simulink model "Parallel_Force_Position_Control"  (R2020b)
settings: Solver=VariableStepAuto  StartTime=0.0  StopTime=20  RelTol=1e-3
values from neighbouring files (symbols this model uses):
  B = myRobot.B_Lagrangian    [hw15_main.m]
  C = myRobot.C_Lagrangian    [hw15_main.m]
  dJ = dJ(1:3  ,:)    [hw15_main.m]
  F = myRobot.F    [hw15_main.m]
  fd = [0;1;0]    [hw15_main.m]
  G = myRobot.G_Lagrangian    [hw15_main.m]
  J_inv = pinv(J)    [hw15_main.m]
  Ja = Ja(1:3,:)    [hw15_main.m]
  K = diag([1 1 1])    [hw15_main.m]
  Kd = diag([1 20 1])    [hw15_main.m]
  Kf = diag([1 10 1]).*10    [hw15_main.m]
  Ki = diag([1 10 1])    [hw15_main.m]
  Kp = diag([1 0.5 1])    [hw15_main.m]
  Md = diag([1 1 1])    [hw15_main.m]
  Md_inv = pinv(Md)    [hw15_main.m]
  xd = [0.3;0;0.1]    [hw15_main.m]
  xr = [0;0.3;0]    [hw15_main.m]
settings Model: Creator=nicol  LastModifiedBy=nicol

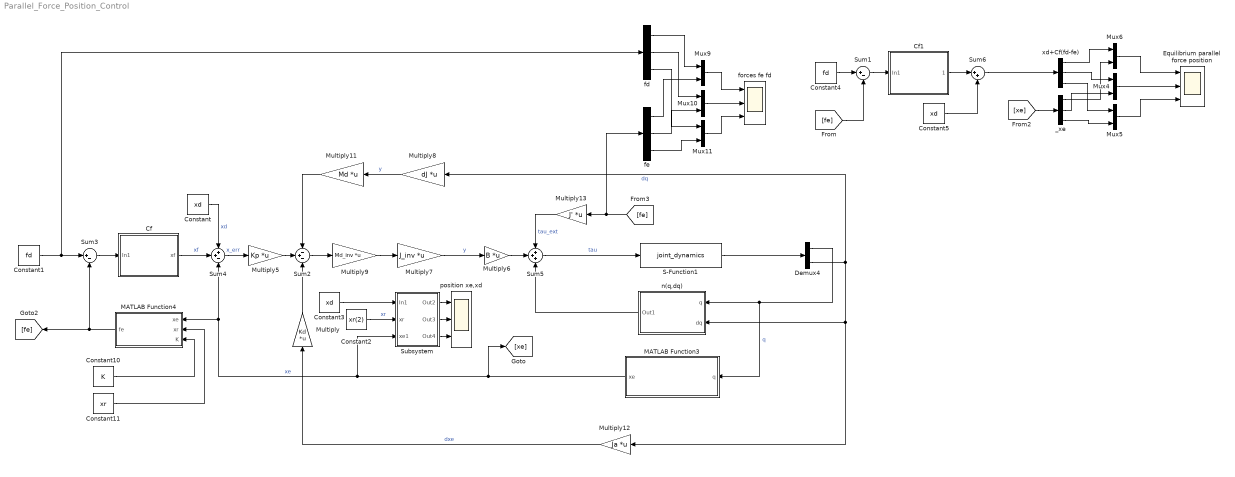
== system Parallel_Force_Position_Control ==
  Cf : Subsystem
  Cf1 : Subsystem
  Constant : Constant  Value=xd
  Constant1 : Constant  Value=fd
  Constant10 : Constant  Value=K
  Constant11 : Constant  Value=xr
  Constant2 : Constant  Value=xr(2)
  Constant3 : Constant  Value=xd
  Constant4 : Constant  Value=fd
  Constant5 : Constant  Value=xd
  Demux4 : Demux  Outputs=2
  Equilibrium parallel force position : Scope  NumInputPorts=3
  MATLAB Function3 : MATLAB Function  TreatAsAtomicUnit=on
  MATLAB Function4 : MATLAB Function  TreatAsAtomicUnit=on
  Multiply : Gain  Gain=Kd  Multiplication=Matrix(K*u)
  Multiply11 : Gain  Gain=Md  Multiplication=Matrix(K*u)
  Multiply12 : Gain  Gain=Ja  Multiplication=Matrix(K*u)
  Multiply13 : Gain  Gain=J'  Multiplication=Matrix(K*u)
  Multiply5 : Gain  Gain=Kp  Multiplication=Matrix(K*u)
  Multiply6 : Gain  Gain=B  Multiplication=Matrix(K*u)
  Multiply7 : Gain  Gain=J_inv  Multiplication=Matrix(K*u)
  Multiply8 : Gain  Gain=dJ  Multiplication=Matrix(K*u)
  Multiply9 : Gain  Gain=Md_inv  Multiplication=Matrix(K*u)
  Mux{4..6,9..11} (6 alike) : Mux  Inputs=2
  S-Function1 : S-Function  FunctionName=joint_dynamics  Parameters=myRobot  SFunctionDeploymentMode=off  EnableBusSupport=off
  Subsystem : Subsystem
  Sum1 : Sum  Inputs=|+-
  Sum2 : Sum  Inputs=-+-
  Sum3 : Sum  Inputs=|+-
  Sum4 : Sum  Inputs=++-
  Sum5 : Sum  Inputs=+++
  Sum6 : Sum  Inputs=|++
  _xe : Demux  Outputs=3
  fd : Demux  Outputs=3
  fe : Demux  Outputs=3
  forces fe fd : Scope  NumInputPorts=3
  n(q,dq) : Subsystem
  position xe,xd : Scope  NumInputPorts=3
  xd+Cf(fd-fe) : Demux  Outputs=3
  wires:
  Sum4/1 -> Multiply5/1  "x_err"
  Multiply/1 -> Sum2/3
  Sum2/1 -> Multiply9/1
  Multiply6/1 -> Sum5/2
  Multiply5/1 -> Sum2/2
  Multiply7/1 -> Multiply6/1  "y"
  Multiply11/1 -> Sum2/1
  Multiply8/1 -> Multiply11/1  "y"
  Multiply9/1 -> Multiply7/1
  Sum5/1 -> S-Function1/1  "tau"
  n(q,dq)/1(Out1) -> Sum5/3
  Demux4/2 -> Multiply8/1, Multiply12/1, n(q,dq)/2(dq)  "dq"
  S-Function1/1 -> Demux4/1
  Multiply12/1 -> Multiply/1  "dxe"
  MATLAB Function3/1(xe) -> [xe], Subsystem/3(xe1), Sum4/3, MATLAB Function4/1(xe)  "xe"
  Constant1/1 -> fd/1, Sum3/1
  MATLAB Function4/1(fe) -> [fe], Sum3/2
  Constant11/1 -> MATLAB Function4/2(xr)
  Constant10/1 -> MATLAB Function4/3(K)
  Demux4/1 -> MATLAB Function3/1(q), n(q,dq)/1(q)  "q"
  Multiply13/1 -> Sum5/1  "tau_ext"
  Cf/1(xf) -> Sum4/2  "xf"
  [fe] -> fe/1, Multiply13/1
  Mux9/1 -> forces fe fd/1
  Mux11/1 -> forces fe fd/3
  fd/2 -> Mux10/1
  Mux10/1 -> forces fe fd/2
  fe/2 -> Mux10/2
  fe/1 -> Mux9/2
  fd/3 -> Mux11/1
  fe/3 -> Mux11/2
  fd/1 -> Mux9/1
  Sum3/1 -> Cf/1(In1)
  Constant/1 -> Sum4/1  "xd"
  Constant4/1 -> Sum1/1
  Sum1/1 -> Cf1/1(In1)
  Cf1/1(" ") -> Sum6/1
  Constant5/1 -> Sum6/2
  Sum6/1 -> xd+Cf(fd-fe)/1
  Mux6/1 -> Equilibrium parallel force position/1
  Mux5/1 -> Equilibrium parallel force position/3
  xd+Cf(fd-fe)/1 -> Mux6/1
  [xe] -> _xe/1
  xd+Cf(fd-fe)/3 -> Mux5/1
  _xe/1 -> Mux6/2
  _xe/2 -> Mux4/2
  _xe/3 -> Mux5/2
  xd+Cf(fd-fe)/2 -> Mux4/1
  Mux4/1 -> Equilibrium parallel force position/2
  [fe] -> Sum1/2
  Constant3/1 -> Subsystem/1(In1)
  Constant2/1 -> Subsystem/2(xr)  "xr"
  Subsystem/1(Out2) -> position xe,xd/1
  Subsystem/2(Out3) -> position xe,xd/2
  Subsystem/3(Out4) -> position xe,xd/3

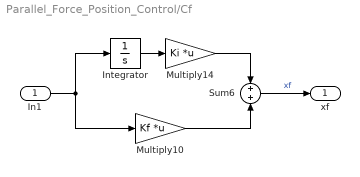
== system Parallel_Force_Position_Control/Cf ==
  In1 : Inport
  Integrator : Integrator
  Multiply10 : Gain  Gain=Kf  Multiplication=Matrix(K*u)
  Multiply14 : Gain  Gain=Ki  Multiplication=Matrix(K*u)
  Sum6 : Sum
  xf : Outport
  wires:
  Multiply14/1 -> Sum6/1
  Integrator/1 -> Multiply14/1
  In1/1 -> Integrator/1, Multiply10/1
  Multiply10/1 -> Sum6/2
  Sum6/1 -> xf/1  "xf"

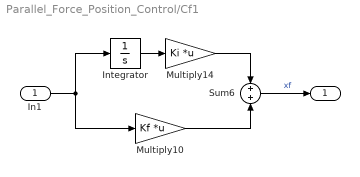
== system Parallel_Force_Position_Control/Cf1 ==
  In1 : Inport
  Integrator : Integrator
  Multiply10 : Gain  Gain=Kf  Multiplication=Matrix(K*u)
  Multiply14 : Gain  Gain=Ki  Multiplication=Matrix(K*u)
  Sum6 : Sum
  " " : Outport
  wires:
  Multiply14/1 -> Sum6/1
  Integrator/1 -> Multiply14/1
  In1/1 -> Integrator/1, Multiply10/1
  Multiply10/1 -> Sum6/2
  Sum6/1 -> " "/1  "xf"

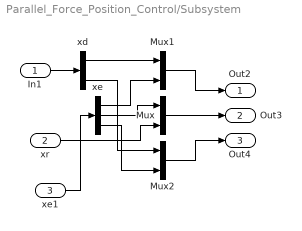
== system Parallel_Force_Position_Control/Subsystem ==
  In1 : Inport
  xr : Inport  Port=2
  xe1 : Inport  Port=3
  Mux : Mux  Inputs=2
  Mux1 : Mux  Inputs=2
  Mux2 : Mux  Inputs=2
  xd : Demux  Outputs=3
  xe : Demux  Outputs=3
  Out2 : Outport
  Out3 : Outport  Port=2
  Out4 : Outport  Port=3
  wires:
  xe/2 -> Mux/1
  xe/3 -> Mux2/2
  xe/1 -> Mux1/2
  xe1/1 -> xe/1
  Mux/1 -> Out3/1
  Mux1/1 -> Out2/1
  xd/1 -> Mux1/1
  xd/3 -> Mux2/1
  Mux2/1 -> Out4/1
  In1/1 -> xd/1
  xr/1 -> Mux/2

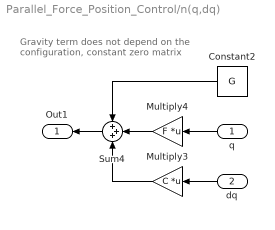
== system Parallel_Force_Position_Control/n(q,dq) ==
  note: Gravity term does not depend on the
      |  configuration, constant zero matrix
  q : Inport
  dq : Inport  Port=2
  Constant2 : Constant  Value=G  VectorParams1D=off
  Multiply3 : Gain  Gain=C  Multiplication=Matrix(K*u)
  Multiply4 : Gain  Gain=F  Multiplication=Matrix(K*u)
  Sum4 : Sum  Inputs=+++
  Out1 : Outport
  wires:
  Sum4/1 -> Out1/1
  Multiply3/1 -> Sum4/3
  Multiply4/1 -> Sum4/2
  Constant2/1 -> Sum4/1
  q/1 -> Multiply4/1
  dq/1 -> Multiply3/1

== matlab function Parallel_Force_Position_Control/MATLAB Function4 ==
  data: xe input; fe output; xr input; K input
function fe = getFe(xe,xr,K)
if(xe(2,1)-xr(2,1)>0)
    fe=K*(xe-xr);
    fe(1)=0;
    fe(3)=0;
else
    fe=zeros(3,1);
end

== matlab function Parallel_Force_Position_Control/MATLAB Function3 ==
  data: q input size=3; xe output size=3
function xe = directKinematics(q)
xe=[ q(1) + 1/5;
    q(3) + 1/5;
    q(2) + 1251/5000]
end
